simulink model "Pendulum"  (R2026a)
settings: Solver=VariableStepAuto  MaxStep=0.001
model workspace (MAT data in the model file):
  b = 0.1
  g = 9.81
  l = 0.5
  m = 0.2

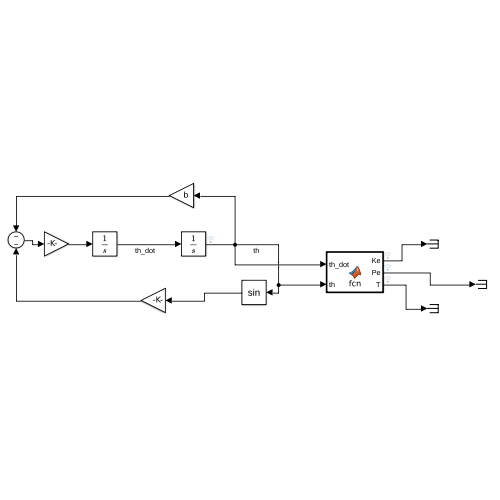
[thumbnail: Simulink's stored preview of the top-level diagram]
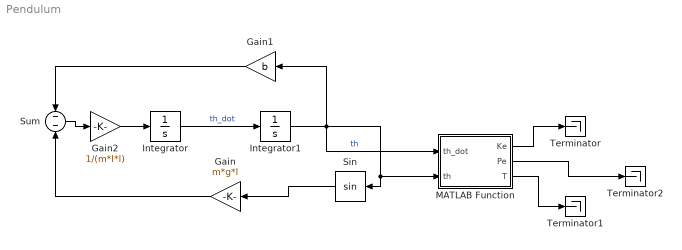
== system Pendulum ==
  Gain : Gain  Gain=m*g*l
  Gain1 : Gain  Gain=b
  Gain2 : Gain  Gain=1/(m*l*l)
  Integrator : Integrator
  Integrator1 : Integrator  InitialCondition=0.5
  MATLAB Function : MATLAB Function  TreatAsAtomicUnit=on
  Sin : Trigonometry
  Sum : Sum  Inputs=-|-
  Terminator : Terminator
  Terminator1 : Terminator
  Terminator2 : Terminator
  wires:
  Integrator/1 -> Integrator1/1  "th_dot"
  Sin/1 -> Gain/1
  Integrator1/1 -> Gain1/1, MATLAB Function/1(th_dot), MATLAB Function/2(th), Sin/1  "th"
  Gain/1 -> Sum/2
  Gain1/1 -> Sum/1
  Sum/1 -> Gain2/1
  Gain2/1 -> Integrator/1
  MATLAB Function/1(Ke) -> Terminator/1
  MATLAB Function/2(Pe) -> Terminator2/1
  MATLAB Function/3(T) -> Terminator1/1

== matlab function Pendulum/MATLAB Function ==
  data: Ke output; Pe output; T output; th_dot input; th input; m parameter; g parameter; l parameter
function [Ke,Pe, T] = fcn(th_dot, th, m, g, l)

Ke = 0.5*m*l*l*th_dot*th_dot;
Pe = m*g*l*(1-cos(th));
T = Ke + Pe;
